simulink subsystem "CiEngine"  (R2025b)
settings: Solver=VariableStepAuto  StartTime=0.0  StopTime=10.0  RelTol=1e-3
undefined symbols (not defined in the file): PlntEngAccPwrTbl, PlntEngAccSpdBpt, PlntEngTimeCECP, PlntEngTimeCEGR, PlntEngTimeCETC, PlntEngTimeCICP, PlntEngTimeCIRL, PlntEngTimeCIVL, PlntEngTimeCVCR, PlntEngTimeCVGT, PlntEngTimeCWGA, PlntEngTimeCWVA
libraries: autolibpowerinfoutils x1, autolibutils x1
settings Model: ModifiedByFormat=The MathWorks, Inc.  Creator=The MathWorks, Inc.  LastModifiedBy=The MathWorks, Inc.
settings SolverCC: MaxZcPerStep=1.0
settings DebuggingCC: UnconnectedInputMsg=warning  UnconnectedOutputMsg=warning  UnconnectedLineMsg=warning
settings ModelReferenceCC: EnableRefExpFcnMdlSchedulingChecks=on
settings RTWCC: GPUComputeCapability=3.5  DLArmComputeVersion=19.05

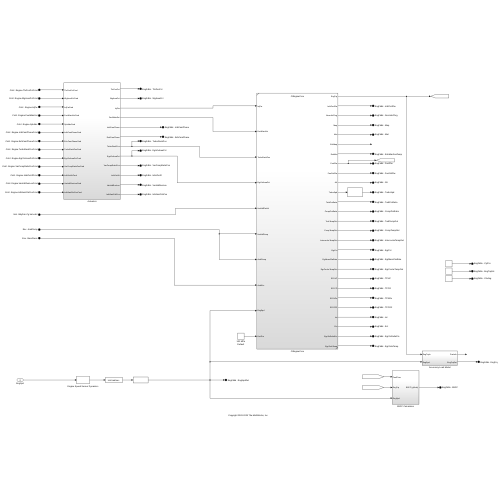
[thumbnail: Simulink's stored preview of the top-level diagram]
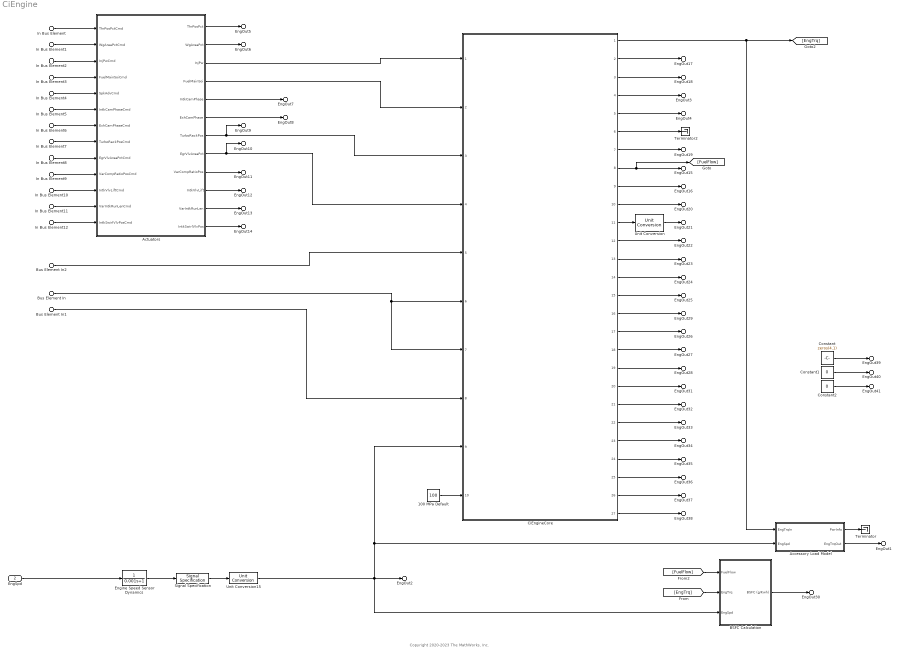
== system CiEngine ==
  note: Copyright 2020-2023 The MathWorks, Inc.
  In Bus Element : Inport  PortName=Cntrl  Element=Engine.ThrPosPctCmd
  In Bus Element1 : Inport  PortName=Cntrl  Element=Engine.WgAreaPctCmd
  In Bus Element2 : Inport  PortName=Cntrl  Element=Engine.InjPw
  In Bus Element3 : Inport  PortName=Cntrl  Element=Engine.FuelMainSoi
  In Bus Element4 : Inport  PortName=Cntrl  Element=Engine.SpkAdv
  In Bus Element5 : Inport  PortName=Cntrl  Element=Engine.IntkCamPhaseCmd
  In Bus Element6 : Inport  PortName=Cntrl  Element=Engine.ExhCamPhaseCmd
  In Bus Element7 : Inport  PortName=Cntrl  Element=Engine.TurboRackPosCmd
  In Bus Element8 : Inport  PortName=Cntrl  Element=Engine.EgrVlvAreaPctCmd
  In Bus Element9 : Inport  PortName=Cntrl  Element=Engine.VarCompRatioPosCmd
  In Bus Element10 : Inport  PortName=Cntrl  Element=Engine.IntkVlvLiftCmd
  In Bus Element11 : Inport  PortName=Cntrl  Element=Engine.VarIntkRunLenCmd
  In Bus Element12 : Inport  PortName=Cntrl  Element=Engine.IntkSwirlVlvPosCmd
  EngSpd : Inport  Port=2  Unit=rad/sec
  Bus Element In : Inport  Port=3  PortName=Env  Element=AmbTemp
  Bus Element In1 : Inport  Port=3  PortName=Env  Element=BaroPress
  Bus Element In2 : Inport  Port=4  PortName=Veh  Element=BdyFrm.Cg.Vel.xdot
  100 MPa Default : Constant  Value=100  SampleTime=-1
  Accessory Load Model : Subsystem
  Actuators : Subsystem
  BSFC Calculation : Subsystem
  CiEngineCore : Subsystem  ReferencedSubsystem=CiEngineCore
  Constant : Constant  Value=zeros(4,1)  SampleTime=-1
  Constant1 : Constant  Value=0  SampleTime=-1
  Constant2 : Constant  Value=0  SampleTime=-1
  Engine Speed Sensor Dynamics : TransferFcn  Denominator=[0.001 1]
  Signal Specification : SignalSpecification  Unit=rad/sec
  Terminator : Terminator
  Terminator2 : Terminator
  Unit Conversion : UnitConversion
  Unit Conversion15 : UnitConversion
  EngOut1 : Outport  PortName=EngFdbk  Element=EngTrq
  EngOut2 : Outport  PortName=EngFdbk  Element=EngSpdOut
  EngOut3 : Outport  PortName=EngFdbk  Element=Map
  EngOut4 : Outport  PortName=EngFdbk  Element=Mat
  EngOut5 : Outport  PortName=EngFdbk  Element=ThrPosPct
  EngOut6 : Outport  PortName=EngFdbk  Element=WgAreaPct
  EngOut7 : Outport  PortName=EngFdbk  Element=IntkCamPhase
  EngOut8 : Outport  PortName=EngFdbk  Element=ExhCamPhase
  EngOut9 : Outport  PortName=EngFdbk  Element=TurboRackPos
  EngOut10 : Outport  PortName=EngFdbk  Element=EgrVlvAreaPct
  EngOut11 : Outport  PortName=EngFdbk  Element=VarCompRatioPos
  EngOut12 : Outport  PortName=EngFdbk  Element=IntkVlvLift
  EngOut13 : Outport  PortName=EngFdbk  Element=VarIntkRunLen
  EngOut14 : Outport  PortName=EngFdbk  Element=IntkSwirlVlvPos
  EngOut15 : Outport  PortName=EngFdbk  Element=FuelFlw
  EngOut16 : Outport  PortName=EngFdbk  Element=FuelVolFlw
  EngOut17 : Outport  PortName=EngFdbk  Element=IntkPortFlw
  EngOut18 : Outport  PortName=EngFdbk  Element=NormAirChrg
  EngOut19 : Outport  PortName=EngFdbk  Element=ExhManGasTemp
  EngOut20 : Outport  PortName=EngFdbk  Element=Afr
  EngOut21 : Outport  PortName=EngFdbk  Element=TurboSpd
  EngOut22 : Outport  PortName=EngFdbk  Element=TurbPrsRatio
  EngOut23 : Outport  PortName=EngFdbk  Element=CompPrsRatio
  EngOut24 : Outport  PortName=EngFdbk  Element=TurbTempOut
  EngOut25 : Outport  PortName=EngFdbk  Element=CompTempOut
  EngOut26 : Outport  PortName=EngFdbk  Element=EgrPct
  EngOut27 : Outport  PortName=EngFdbk  Element=EgrMassFlwRate
  EngOut28 : Outport  PortName=EngFdbk  Element=EgrCoolerTempOut
  EngOut29 : Outport  PortName=EngFdbk  Element=IntercoolerTempOut
  EngOut30 : Outport  PortName=EngFdbk  Element=BSFC
  EngOut31 : Outport  PortName=EngFdbk  Element=TPHC
  EngOut32 : Outport  PortName=EngFdbk  Element=TPCO
  EngOut33 : Outport  PortName=EngFdbk  Element=TPNOx
  EngOut34 : Outport  PortName=EngFdbk  Element=TPCO2
  EngOut35 : Outport  PortName=EngFdbk  Element=Iat
  EngOut36 : Outport  PortName=EngFdbk  Element=Ect
  EngOut37 : Outport  PortName=EngFdbk  Element=EgrVlvDeltaPrs
  EngOut38 : Outport  PortName=EngFdbk  Element=EgrVlvInTemp
  EngOut39 : Outport  PortName=EngFdbk  Element=CylPrs
  EngOut40 : Outport  PortName=EngFdbk  Element=EngTrqCrk
  EngOut41 : Outport  PortName=EngFdbk  Element=CrkAng
  wires:
  Accessory Load Model/2(EngTrqOut) -> EngOut1/1
  Constant2/1 -> EngOut41/1
  Actuators/2(WgAreaPct) -> EngOut6/1
  100 MPa Default/1 -> CiEngineCore/10
  Bus Element In1/1 -> CiEngineCore/8
  Actuators/12(IntkSwirlVlvPos) -> EngOut14/1
  Accessory Load Model/1(PwrInfo) -> Terminator/1
  CiEngineCore/25 -> EngOut36/1
  CiEngineCore/17 -> EngOut26/1
  Constant/1 -> EngOut39/1
  CiEngineCore/24 -> EngOut35/1
  CiEngineCore/8 -> [FuelFlow], EngOut15/1
  CiEngineCore/9 -> EngOut16/1
  CiEngineCore/27 -> EngOut38/1
  Constant1/1 -> EngOut40/1
  CiEngineCore/20 -> EngOut31/1
  CiEngineCore/5 -> EngOut4/1
  CiEngineCore/21 -> EngOut32/1
  CiEngineCore/16 -> EngOut29/1
  CiEngineCore/26 -> EngOut37/1
  CiEngineCore/14 -> EngOut24/1
  CiEngineCore/12 -> EngOut22/1
  CiEngineCore/10 -> EngOut20/1
  CiEngineCore/7 -> EngOut19/1
  CiEngineCore/1 -> Accessory Load Model/1(EngTrqIn), [EngTrq]
  CiEngineCore/4 -> EngOut3/1
  CiEngineCore/15 -> EngOut25/1
  Actuators/7(TurboRackPos) -> EngOut9/1, CiEngineCore/3
  Actuators/4(FuelMainSoi) -> CiEngineCore/2
  CiEngineCore/3 -> EngOut18/1
  CiEngineCore/13 -> EngOut23/1
  Actuators/11(VarIntkRunLen) -> EngOut13/1
  BSFC Calculation/1(BSFC (g/Kwh)) -> EngOut30/1
  Bus Element In/1 -> CiEngineCore/7, CiEngineCore/6
  [EngTrq] -> BSFC Calculation/2(EngTrq)
  CiEngineCore/2 -> EngOut17/1
  CiEngineCore/18 -> EngOut27/1
  Actuators/10(IntkVlvLift) -> EngOut12/1
  Actuators/3(InjPw) -> CiEngineCore/1
  Actuators/8(EgrVlvAreaPct) -> EngOut10/1, CiEngineCore/4
  Actuators/5(IntkCamPhase) -> EngOut7/1
  CiEngineCore/23 -> EngOut34/1
  Actuators/9(VarCompRatioPos) -> EngOut11/1
  Bus Element In2/1 -> CiEngineCore/5
  Actuators/6(ExhCamPhase) -> EngOut8/1
  CiEngineCore/19 -> EngOut28/1
  [FuelFlow] -> BSFC Calculation/1(FuelFlow)
  Unit Conversion15/1 -> BSFC Calculation/3(EngSpd), EngOut2/1, Accessory Load Model/2(EngSpd), CiEngineCore/9
  Actuators/1(ThrPosPct) -> EngOut5/1
  CiEngineCore/22 -> EngOut33/1
  In Bus Element11/1 -> Actuators/12(VarIntkRunLenCmd)
  In Bus Element10/1 -> Actuators/11(IntkVlvLiftCmd)
  In Bus Element7/1 -> Actuators/8(TurboRackPosCmd)
  In Bus Element8/1 -> Actuators/9(EgrVlvAreaPctCmd)
  In Bus Element5/1 -> Actuators/6(IntkCamPhaseCmd)
  In Bus Element6/1 -> Actuators/7(ExhCamPhaseCmd)
  In Bus Element/1 -> Actuators/1(ThrPosPctCmd)
  In Bus Element1/1 -> Actuators/2(WgAreaPctCmd)
  In Bus Element9/1 -> Actuators/10(VarCompRatioPosCmd)
  In Bus Element3/1 -> Actuators/4(FuelMainSoiCmd)
  In Bus Element12/1 -> Actuators/13(IntkSwirlVlvPosCmd)
  In Bus Element4/1 -> Actuators/5(SpkAdvCmd)
  In Bus Element2/1 -> Actuators/3(InjPwCmd)
  CiEngineCore/6 -> Terminator2/1
  CiEngineCore/11 -> Unit Conversion/1
  Unit Conversion/1 -> EngOut21/1
  Signal Specification/1 -> Unit Conversion15/1
  Engine Speed Sensor Dynamics/1 -> Signal Specification/1
  EngSpd/1 -> Engine Speed Sensor Dynamics/1

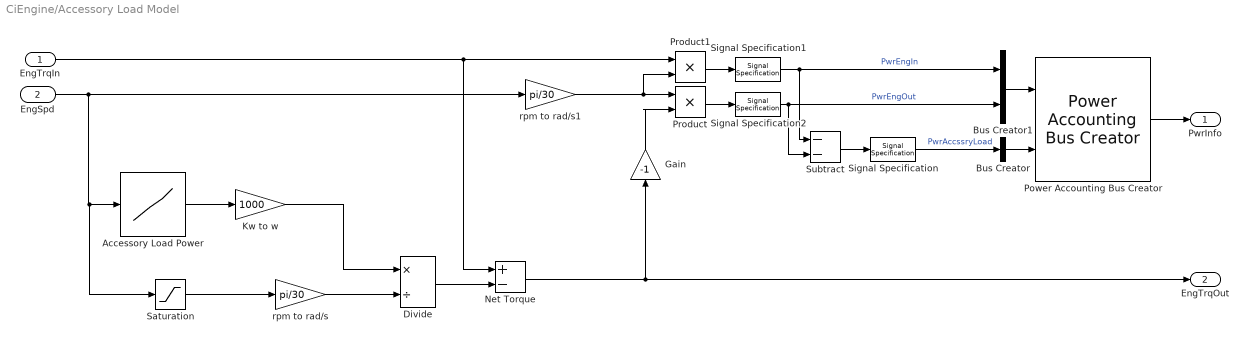
== system CiEngine/Accessory Load Model ==
  EngTrqIn : Inport
  EngSpd : Inport  Port=2
  Accessory Load Power : Lookup_n-D  NumberOfTableDimensions=1  LookupTableObject=''  BreakpointsForDimension1=PlntEngAccSpdBpt  Table=PlntEngAccPwrTbl  ExtrapMethod=Clip  InternalRulePriority=Speed  RndMeth=Simplest
  Bus Creator : BusCreator  Inputs=1
  Bus Creator1 : BusCreator  Inputs=2
  Divide : Product  Inputs=*/
  Gain : Gain  Gain=-1
  Kw to w : Gain  Gain=1000
  Net Torque : Sum  Inputs=+-
  Power Accounting Bus Creator : autolibpowerinfoutils/Power Accounting Bus Creator  AssctBlkSelPopup=Parent  RefBlkName='libraryname/blkname'  PwrTrnsfrdCheckBox=on  PwrNotTrnsfrdCheckBox=on  PwrStoredCheckBox=off  aMode=aMode
  Product : Product
  Product1 : Product
  Saturation : Saturate  UpperLimit=Inf  LowerLimit=300
  Signal Specification : SignalSpecification  Unit=W
  Signal Specification1 : SignalSpecification  Unit=W
  Signal Specification2 : SignalSpecification  Unit=W
  Subtract : Sum  Inputs=--
  rpm to rad/s : Gain  Gain=pi/30
  rpm to rad/s1 : Gain  Gain=pi/30
  PwrInfo : Outport  VectorParamsAs1DForOutWhenUnconnected=off
  EngTrqOut : Outport  Port=2  Unit=N*m  VectorParamsAs1DForOutWhenUnconnected=off
  wires:
  Divide/1 -> Net Torque/2
  Accessory Load Power/1 -> Kw to w/1
  EngSpd/1 -> Saturation/1, Accessory Load Power/1, rpm to rad/s1/1
  Saturation/1 -> rpm to rad/s/1
  rpm to rad/s/1 -> Divide/2
  Net Torque/1 -> EngTrqOut/1, Gain/1
  Bus Creator/1 -> Power Accounting Bus Creator/2
  Kw to w/1 -> Divide/1
  Bus Creator1/1 -> Power Accounting Bus Creator/1
  EngTrqIn/1 -> Product1/1, Net Torque/1
  Subtract/1 -> Signal Specification/1
  Signal Specification/1 -> Bus Creator/1  "PwrAccssryLoad"
  Power Accounting Bus Creator/1 -> PwrInfo/1
  Product/1 -> Signal Specification2/1
  Product1/1 -> Signal Specification1/1
  rpm to rad/s1/1 -> Product1/2, Product/1
  Signal Specification1/1 -> Subtract/1, Bus Creator1/1  "PwrEngIn"
  Signal Specification2/1 -> Subtract/2, Bus Creator1/2  "PwrEngOut"
  Gain/1 -> Product/2

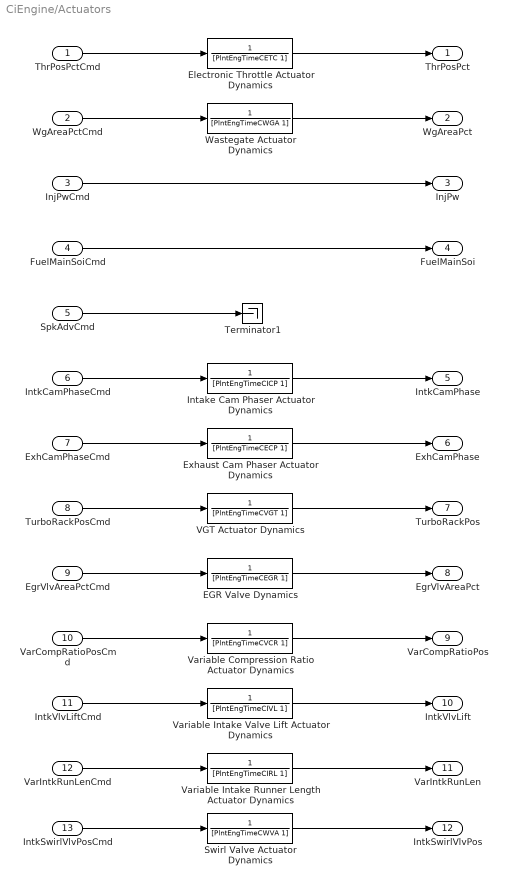
== system CiEngine/Actuators ==
  ThrPosPctCmd : Inport  Unit=%
  WgAreaPctCmd : Inport  Port=2  Unit=%
  InjPwCmd : Inport  Port=3  Unit=ms
  FuelMainSoiCmd : Inport  Port=4  Unit=deg
  SpkAdvCmd : Inport  Port=5  Unit=deg
  IntkCamPhaseCmd : Inport  Port=6  Unit=deg
  ExhCamPhaseCmd : Inport  Port=7  Unit=deg
  TurboRackPosCmd : Inport  Port=8  Unit=1
  EgrVlvAreaPctCmd : Inport  Port=9  Unit=%
  VarCompRatioPosCmd : Inport  Port=10
  IntkVlvLiftCmd : Inport  Port=11
  VarIntkRunLenCmd : Inport  Port=12
  IntkSwirlVlvPosCmd : Inport  Port=13
  EGR Valve Dynamics : TransferFcn  Denominator=[PlntEngTimeCEGR 1]
  Electronic Throttle Actuator Dynamics : TransferFcn  Denominator=[PlntEngTimeCETC 1]
  Exhaust Cam Phaser Actuator Dynamics : TransferFcn  Denominator=[PlntEngTimeCECP 1]
  Intake Cam Phaser Actuator Dynamics : TransferFcn  Denominator=[PlntEngTimeCICP 1]
  Swirl Valve Actuator Dynamics : TransferFcn  Denominator=[PlntEngTimeCWVA 1]
  Terminator1 : Terminator
  VGT Actuator Dynamics : TransferFcn  Denominator=[PlntEngTimeCVGT 1]
  Variable Compression Ratio Actuator Dynamics : TransferFcn  Denominator=[PlntEngTimeCVCR 1]
  Variable Intake Runner Length Actuator Dynamics : TransferFcn  Denominator=[PlntEngTimeCIRL 1]
  Variable Intake Valve Lift Actuator Dynamics : TransferFcn  Denominator=[PlntEngTimeCIVL 1]
  Wastegate Actuator Dynamics : TransferFcn  Denominator=[PlntEngTimeCWGA 1]
  ThrPosPct : Outport  Unit=%  VectorParamsAs1DForOutWhenUnconnected=off
  WgAreaPct : Outport  Port=2  Unit=%  VectorParamsAs1DForOutWhenUnconnected=off
  InjPw : Outport  Port=3  VectorParamsAs1DForOutWhenUnconnected=off
  FuelMainSoi : Outport  Port=4  VectorParamsAs1DForOutWhenUnconnected=off
  IntkCamPhase : Outport  Port=5  Unit=deg  VectorParamsAs1DForOutWhenUnconnected=off
  ExhCamPhase : Outport  Port=6  Unit=deg  VectorParamsAs1DForOutWhenUnconnected=off
  TurboRackPos : Outport  Port=7  Unit=1  VectorParamsAs1DForOutWhenUnconnected=off
  EgrVlvAreaPct : Outport  Port=8  Unit=%  VectorParamsAs1DForOutWhenUnconnected=off
  VarCompRatioPos : Outport  Port=9  VectorParamsAs1DForOutWhenUnconnected=off
  IntkVlvLift : Outport  Port=10  VectorParamsAs1DForOutWhenUnconnected=off
  VarIntkRunLen : Outport  Port=11  VectorParamsAs1DForOutWhenUnconnected=off
  IntkSwirlVlvPos : Outport  Port=12  VectorParamsAs1DForOutWhenUnconnected=off
  wires:
  Variable Compression Ratio Actuator Dynamics/1 -> VarCompRatioPos/1
  Variable Intake Valve Lift Actuator Dynamics/1 -> IntkVlvLift/1
  Variable Intake Runner Length Actuator Dynamics/1 -> VarIntkRunLen/1
  Swirl Valve Actuator Dynamics/1 -> IntkSwirlVlvPos/1
  Intake Cam Phaser Actuator Dynamics/1 -> IntkCamPhase/1
  Exhaust Cam Phaser Actuator Dynamics/1 -> ExhCamPhase/1
  Wastegate Actuator Dynamics/1 -> WgAreaPct/1
  Electronic Throttle Actuator Dynamics/1 -> ThrPosPct/1
  FuelMainSoiCmd/1 -> FuelMainSoi/1
  IntkVlvLiftCmd/1 -> Variable Intake Valve Lift Actuator Dynamics/1
  IntkSwirlVlvPosCmd/1 -> Swirl Valve Actuator Dynamics/1
  WgAreaPctCmd/1 -> Wastegate Actuator Dynamics/1
  ThrPosPctCmd/1 -> Electronic Throttle Actuator Dynamics/1
  ExhCamPhaseCmd/1 -> Exhaust Cam Phaser Actuator Dynamics/1
  IntkCamPhaseCmd/1 -> Intake Cam Phaser Actuator Dynamics/1
  VarCompRatioPosCmd/1 -> Variable Compression Ratio Actuator Dynamics/1
  VarIntkRunLenCmd/1 -> Variable Intake Runner Length Actuator Dynamics/1
  InjPwCmd/1 -> InjPw/1
  VGT Actuator Dynamics/1 -> TurboRackPos/1
  EGR Valve Dynamics/1 -> EgrVlvAreaPct/1
  TurboRackPosCmd/1 -> VGT Actuator Dynamics/1
  EgrVlvAreaPctCmd/1 -> EGR Valve Dynamics/1
  SpkAdvCmd/1 -> Terminator1/1

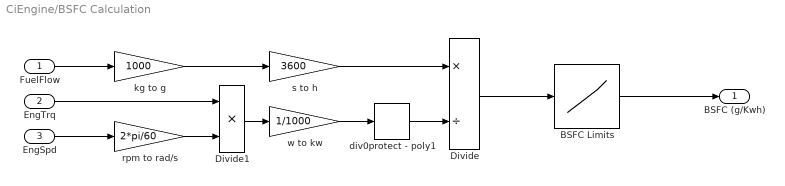
== system CiEngine/BSFC Calculation ==
  FuelFlow : Inport
  EngTrq : Inport  Port=2
  EngSpd : Inport  Port=3
  BSFC Limits : Lookup_n-D  NumberOfTableDimensions=1  BreakpointsForDimension1=[0 500]  Table=[0 500]  ExtrapMethod=Clip  InternalRulePriority=Speed  RndMeth=Simplest
  Divide : Product  Inputs=*/
  Divide1 : Product  Inputs=**
  div0protect - poly1 : autolibutils/div0protect - poly  thresh=1e-6  ZeroCross1=off  aMode=aMode
  kg to g : Gain  Gain=1000
  rpm to rad/s : Gain  Gain=2*pi/60
  s to h : Gain  Gain=3600
  w to kw : Gain  Gain=1/1000
  BSFC (g/Kwh) : Outport  VectorParamsAs1DForOutWhenUnconnected=off
  wires:
  Divide1/1 -> w to kw/1
  kg to g/1 -> s to h/1
  FuelFlow/1 -> kg to g/1
  rpm to rad/s/1 -> Divide1/2
  EngSpd/1 -> rpm to rad/s/1
  EngTrq/1 -> Divide1/1
  Divide/1 -> BSFC Limits/1
  w to kw/1 -> div0protect - poly1/1
  s to h/1 -> Divide/1
  BSFC Limits/1 -> BSFC (g/Kwh)/1
  div0protect - poly1/1 -> Divide/2
